simulink model "Permissable_Charge_Current"  (R2024a)
settings: Solver=VariableStepAuto  StartTime=0.0  StopTime=10000  RelTol=1e-3
undefined symbols (not defined in the file): Ion, Lithium
libraries: spsBatteryLib x2, spsControlledCurrentSourceLib x2, spsVoltageMeasurementLib x2, spspowerguiLib x2, slpidlib x1
settings Model: Creator=ezeki  LastModifiedBy=ezeki

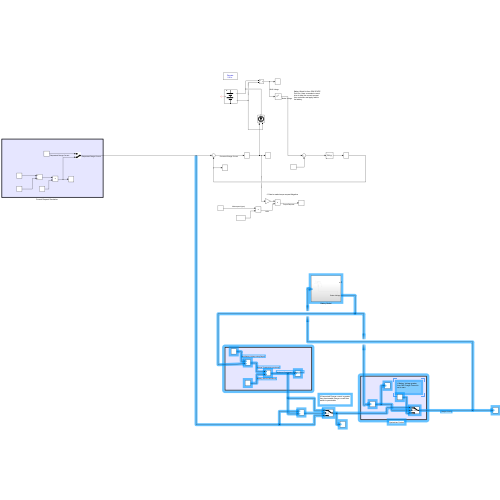
[thumbnail: Simulink's stored preview of the top-level diagram]
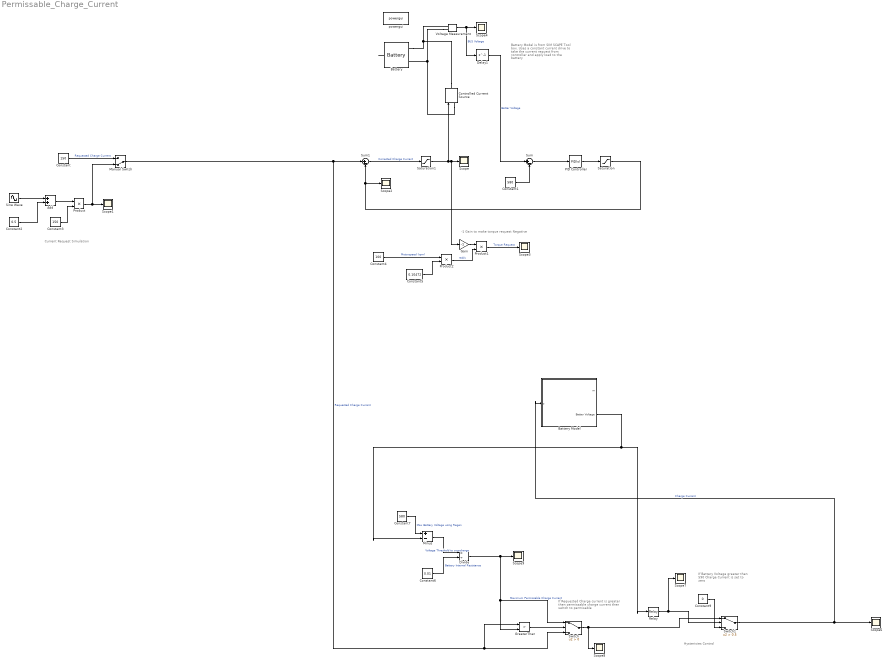
== system Permissable_Charge_Current ==
  note: Hysterisies Control
  note: Current Request Simulation
  note: If Requested Charge current is greater then permissable charge current then switch to permisable
  note: If Battery Voltage greater then 590 Charge Current is set to zero
  note: -1 Gain to make torque request Negative
  note: Battery Model is from SIM SCAPE Tool box. Uses a constant current drive to take the current request from controller and apply load to the battery
  Add : Sum
  Battery : spsBatteryLib/Battery  BatType=Lithium-Ion  ShowTempParam=off  ThermalPreset=no  ShowAgeParam=off  NomV=532.8  NomQ=1152  SOC=85  Batt_Tr=5  PresetModel=on  MaxQ=1152  MinV=399.6  FullV=620.1723  Dis_rate=500.8696  R=0.004625  Normal_OP=1041.8087  expZone="[575.6296      56.59826]"  current=[6.5 13 32.5]  Units=Time  Tci=20  NomT=20  T2=-30  MaxQ2=4.8  FullV2=7.1  Normal_OP2=5.655  expZone2="[6.58           1]"  Rca=0.6  ti=2000  Dp=0  Neq0=0  Tsim=1e6  Ta1=25  Qeol=5.4*0.9  Reol=0.013333*1.2  Char_age=[2.3478, 3]  Dis_age=[2.3478, 10]  N1=1500  N2=10500  N3=1000  N4=1400  Ta2=45  N5=950
  Battery Model : Subsystem
  Constant : Constant  Value=150
  Constant1 : Constant  Value=580
  Constant2 : Constant  Value=0.5
  Constant3 : Constant  Value=150
  Constant4 : Constant  Value=100
  Constant5 : Constant  Value=0.10472
  Constant6 : Constant  Value=0.01
  Constant7 : Constant  Value=580
  Constant9 : Constant  Value=0
  Controlled Current Source : spsControlledCurrentSourceLib/Controlled Current Source  Initialize=on  Source_Type=AC  Amplitude=0  Phase=0  Frequency=0  Measurements=None
  Delay1 : Delay  DelayLength=1  InitialCondition=600
  Divide : Product  Inputs=*/
  Gain : Gain  Gain=-1
  GreaterThan : RelationalOperator  Operator=>  OutDataTypeStr=boolean  RndMeth=Simplest  InputSameDT=off
  Manual Switch : ManualSwitch  CurrentSetting=0
  Minus : Sum  Inputs=+-
  PID Controller : slpidlib/PID Controller  Controller=PID  Form=Parallel  TimeDomain=Continuous-time  UseExternalTs=off  SampleTime=-1  IntegratorMethod=Forward Euler  FilterMethod=Forward Euler  ControllerParametersSource=internal  P=175.021278663276  I=0.0294180003563177  UseKiTs=off  D=-154449.60261899  UseExternalDerivativeSource=off  N=0.00113319345401641  UseFilter=on  TunerSelectOption=Transfer Function Based (PID Tuner App)  InitialConditionSource=internal  InitialConditionForIntegrator=0  InitialConditionForFilter=0  DifferentiatorICPrevScaledInput=0  ExternalReset=none  TrackingMode=off  Kt=1  LimitOutput=off  SatLimitsSource=internal  UpperSaturationLimit=inf  LowerSaturationLimit=-inf  LinearizeAsGain=on  AntiWindupMode=none  Kb=1  LimitIntegrator=off  UpperIntegratorSaturationLimit=inf  LowerIntegratorSaturationLimit=-inf  POutMin=[]  POutMax=[]  IOutMin=[]  IOutMax=[]  DOutMin=[]  DOutMax=[]  NOutMin=[]  NOutMax=[]  SumOutMin=[]  SumOutMax=[]  SaturationOutMin=[]  SaturationOutMax=[]  PParamMin=[]  PParamMax=[]  IParamMin=[]  IParamMax=[]  DParamMin=[]  DParamMax=[]  NParamMin=[]  NParamMax=[]  KbParamMin=[]  KbParamMax=[]  KtParamMin=[]  KtParamMax=[]  KbOutMin=[]  KbOutMax=[]  KtOutMin=[]  KtOutMax=[]  IntegratorOutMin=[]  IntegratorOutMax=[]  FilterOutMin=[]  FilterOutMax=[]  SumI1OutMin=[]  SumI1OutMax=[]  SumI2OutMin=[]  SumI2OutMax=[]  SumI3OutMin=[]  SumI3OutMax=[]  SumI4OutMin=[]  SumI4OutMax=[]  SumDOutMin=[]  SumDOutMax=[]  DifferentiatorOutMin=[]  DifferentiatorOutMax=[]  FilterDiffOutCoefMin=[]  FilterDiffOutCoefMax=[]  ReciprocalOutMin=[]  ReciprocalOutMax=[]  SumDenOutMin=[]  SumDenOutMax=[]  SumNumOutMin=[]  SumNumOutMax=[]  DivideOutMin=[]  DivideOutMax=[]  UdiffTsProdOutMin=[]  UdiffTsProdOutMax=[]  NTsProdOutMin=[]  NTsProdOutMax=[]  UintegralTsProdOutMin=[]  UintegralTsProdOutMax=[]  UngainTsProdOutMin=[]  UngainTsProdOutMax=[]  ClampingZeroOutDataTypeStr=Inherit: Inherit via back propagation  ClampingZeroOutMin=[]  ClampingZeroOutMax=[]  FilterDenConstantOutDataTypeStr=Inherit: Inherit via back propagation  FilterDenConstantOutMin=[]  FilterDenConstantOutMax=[]  PCopyOutDataTypeStr=Inherit: Inherit via back propagation  PCopyOutMin=[]  PCopyOutMax=[]  NCopyOutDataTypeStr=Inherit: Inherit via back propagation  NCopyOutMin=[]  NCopyOutMax=[]  IntegratorContinuousStateAttributes=''  IntegratorStateMustResolveToSignalObject=off  IntegratorRTWStateStorageClass=Auto  FilterContinuousStateAttributes=''  FilterStateMustResolveToSignalObject=off  FilterRTWStateStorageClass=Auto  ParallelPVariant=InternalParameters  IdealPVariant=Disabled  IVariant=InternalParameters  DVariant=InternalParameters  IntegratorVariant=Continuous  SatVariant=Disabled  AWVariant=Passthrough  PCopyVariant=Disabled  TRVariant=Disabled  FdbkBlocksVariant=Forward  IdealPFdbkVariant=Disabled  SatFdbkVariant=Disabled  DerivativeFilterVariant=ContFilter  NVariant=InternalParameters  NCopyVariant=Disabled  FilterICVariant=InternalICsFilter  IntegratorICVariant=InternalICs  ExternalResetVariant=Disabled  TRSumVariant=Passthrough  SumFdbkVariant=Disabled  SumVariant=Sum_PID  TsampFilterVariant=InternalTs  TsampNgainVariant=Passthrough  TsampIntegralVariant=Disabled_SignalSpec  ExternalSaturationOutDataTypeStr=Inherit: Same as second input  DerivativeSourceVariant=ErrorSignal
  Product : Product
  Product1 : Product
  Product2 : Product
  Relay : Relay  OnSwitchValue=590  OffSwitchValue=585  OnOutputValue=0  OffOutputValue=1
  Saturation : Saturate  UpperLimit=150  LowerLimit=0
  Saturation1 : Saturate  UpperLimit=inf  LowerLimit=0
  Scope{,1..4,6..9} (9 alike) : Scope
  Sine Wave : Sin  Amplitude=0.5  Frequency=0.01  SampleTime=0
  Sum : Sum  Inputs=|+-
  Sum1 : Sum  Inputs=|+-
  Switch : Switch  Criteria=u2 > Threshold  SaturateOnIntegerOverflow=off  InputSameDT=off
  Switch1 : Switch  Criteria=u2 > Threshold  Threshold=0.5  SaturateOnIntegerOverflow=off  InputSameDT=off
  Voltage Measurement : spsVoltageMeasurementLib/Voltage Measurement  PhasorSimulation=off  OutputType=Complex  PSBequivalent=0
  powergui : spspowerguiLib/powergui  Priority=1  SimulationMode=Discrete  SampleTime=0.01  frequency=60  Iterations=50  frequencyindice=0  Pbase=100e6  ErrMax=1e-4  UnitsV=kV  UnitsW=MW  buscounter=0  FunctionMessages=off  echomessages=off  EnableUseOfTLC=off  CurrentSourceSwitches=off  DisableSnubberDevices=off  DisableRonSwitches=off  DisableVfSwitches=off  DisplayEquations=off  AutomaticDiscreteSolvers=off  SolverType=Tustin/Backward Euler (TBE)  Interpol=off  ExternalGateDelay=off  methode=off  Ts=100  x0status=blocks  SPID=on  SwTol=0  HookPort=off  NonlinearTolerance=1e-4  nMaxIteration=100  ContinueOnMaxIteration=off  RestoreLinks=warning  ResistiveCurrentMeasurement=off  Frange=[0:2:500]  Ylog=off  Xlog=on  ShowGrid=off  save=off  variable=ZData  structure=0  ZoomFFT=off  StartTime=0.0  cycles=1  DisplayStyle=1  fundamental=60  FreqAxis=off  MaxFrequency=1000  frequencyindicesteady=1  RmsSteady=1  display=off
  wires:
  Sum1/1 -> Saturation1/1  "Corrected Charge Current"
  Voltage Measurement/1 -> Delay1/1, Scope4/1  "BUS Voltage"
  Battery/1 -> ?
  Delay1/1 -> Sum/1  "Batter Voltage"
  Constant1/1 -> Sum/2
  Sum/1 -> PID Controller/1
  Manual Switch/1 -> Switch/3, GreaterThan/1, Sum1/1  "Requested Charge Current"
  PID Controller/1 -> Saturation/1
  Sine Wave/1 -> Add/1
  Constant2/1 -> Add/2
  Product/1 -> Manual Switch/2, Scope1/1
  Add/1 -> Product/1
  Constant3/1 -> Product/2
  Constant/1 -> Manual Switch/1  "Requested Charge Current"
  Saturation/1 -> Scope2/1, Sum1/2
  Saturation1/1 -> Gain/1, Scope/1, Controlled Current Source/1
  Constant4/1 -> Product2/1  "Motorspeed (rpm)"
  Product1/1 -> Scope3/1  "Torque Request"
  Gain/1 -> Product1/1
  Product2/1 -> Product1/2  "rad/s"
  Constant5/1 -> Product2/2
  Switch/1 -> Switch1/1, Scope8/1
  Constant6/1 -> Divide/2  "Battery Internal Resistance"
  Divide/1 -> GreaterThan/2, Switch/1, Scope9/1  "Maximum Permissable Charge Current"
  GreaterThan/1 -> Switch/2
  Constant7/1 -> Minus/1  "Max Battery Voltage using Regen"
  Switch1/1 -> Battery Model/1(s), Scope6/1  "Charge Current"
  Relay/1 -> Switch1/2, Scope7/1
  Constant9/1 -> Switch1/3
  Minus/1 -> Divide/1  "Voltage Threshold to overcharge"
  Battery Model/2(Batter Voltage) -> Minus/2, Relay/1
  connections:
  Controlled Current Source/RConn1 -- Battery/LConn1 -- Voltage Measurement/LConn1
  Voltage Measurement/LConn2 -- Controlled Current Source/LConn1 -- Battery/LConn2

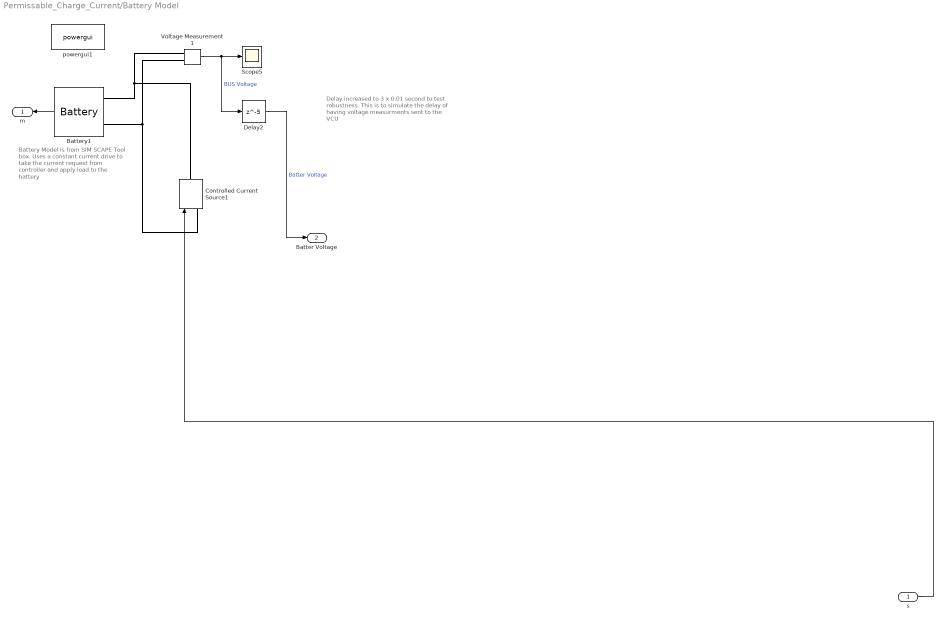
== system Permissable_Charge_Current/Battery Model ==
  note: Delay increased to 3 x 0.01 second to test robustness. This is to simulate the delay of having voltage measurments sent to the VCU
  note: Battery Model is from SIM SCAPE Tool box. Uses a constant current drive to take the current request from controller and apply load to the battery
  s : Inport
  Battery1 : spsBatteryLib/Battery  BatType=Lithium-Ion  ShowTempParam=off  ThermalPreset=no  ShowAgeParam=off  NomV=532.8  NomQ=1152  SOC=85  Batt_Tr=5  PresetModel=on  MaxQ=1152  MinV=399.6  FullV=620.1723  Dis_rate=500.8696  R=0.004625  Normal_OP=1041.8087  expZone="[575.6296      56.59826]"  current=[6.5 13 32.5]  Units=Time  Tci=20  NomT=20  T2=-30  MaxQ2=4.8  FullV2=7.1  Normal_OP2=5.655  expZone2="[6.58           1]"  Rca=0.6  ti=2000  Dp=0  Neq0=0  Tsim=1e6  Ta1=25  Qeol=5.4*0.9  Reol=0.013333*1.2  Char_age=[2.3478, 3]  Dis_age=[2.3478, 10]  N1=1500  N2=10500  N3=1000  N4=1400  Ta2=45  N5=950
  Controlled Current Source1 : spsControlledCurrentSourceLib/Controlled Current Source  Initialize=on  Source_Type=AC  Amplitude=0  Phase=0  Frequency=0  Measurements=None
  Delay2 : Delay  DelayLength=5  InitialCondition=580
  Scope5 : Scope
  Voltage Measurement1 : spsVoltageMeasurementLib/Voltage Measurement  PhasorSimulation=off  OutputType=Complex  PSBequivalent=0
  powergui1 : spspowerguiLib/powergui  Priority=1  SimulationMode=Discrete  SampleTime=0.01  frequency=60  Iterations=50  frequencyindice=0  Pbase=100e6  ErrMax=1e-4  UnitsV=kV  UnitsW=MW  buscounter=0  FunctionMessages=off  echomessages=off  EnableUseOfTLC=off  CurrentSourceSwitches=off  DisableSnubberDevices=off  DisableRonSwitches=off  DisableVfSwitches=off  DisplayEquations=off  AutomaticDiscreteSolvers=off  SolverType=Tustin/Backward Euler (TBE)  Interpol=off  ExternalGateDelay=off  methode=off  Ts=100  x0status=blocks  SPID=on  SwTol=0  HookPort=off  NonlinearTolerance=1e-4  nMaxIteration=100  ContinueOnMaxIteration=off  RestoreLinks=warning  ResistiveCurrentMeasurement=off  Frange=[0:2:500]  Ylog=off  Xlog=on  ShowGrid=off  save=off  variable=ZData  structure=0  ZoomFFT=off  StartTime=0.0  cycles=1  DisplayStyle=1  fundamental=60  FreqAxis=off  MaxFrequency=1000  frequencyindicesteady=1  RmsSteady=1  display=off
  m : Outport
  Batter Voltage : Outport  Port=2
  wires:
  Voltage Measurement1/1 -> Delay2/1, Scope5/1  "BUS Voltage"
  s/1 -> Controlled Current Source1/1
  Delay2/1 -> Batter Voltage/1  "Batter Voltage"
  Battery1/1 -> m/1
  connections:
  Voltage Measurement1/LConn1 -- Controlled Current Source1/RConn1 -- Battery1/LConn1
  Battery1/LConn2 -- Voltage Measurement1/LConn2 -- Controlled Current Source1/LConn1
